simulink subsystem "template_offline_MCP_variant_nlpsol_shared_subsystem"  (R2023b)
settings: Solver=VariableStepAuto  StartTime=0.0  StopTime=10.0  RelTol=1e-3
undefined symbols (not defined in the file): param_MPC1, param_MPC1_traj_data, param_weight_MPC1
settings Model: Creator=emu  LastModifiedBy=emu

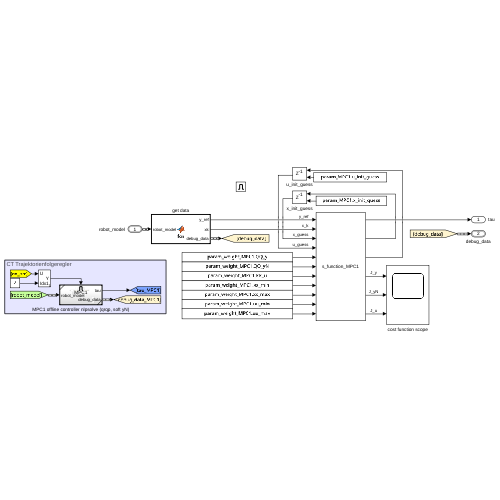
[thumbnail: Simulink's stored preview of the top-level diagram]
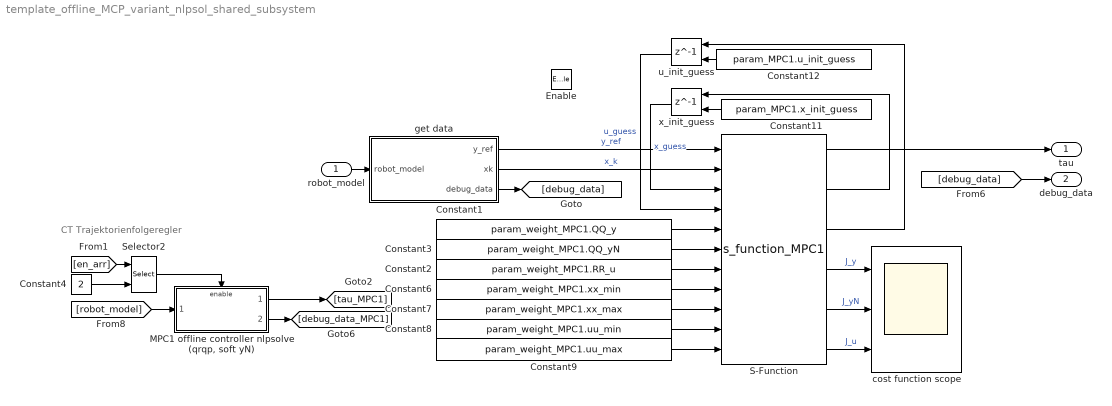
== system template_offline_MCP_variant_nlpsol_shared_subsystem ==
  note: CT Trajektorienfolgeregler
  robot_model : Inport  OutDataTypeStr=Bus: robot_model
  Enable : EnablePort
  Constant1 : Constant  Value=param_weight_MPC1.QQ_y
  Constant11 : Constant  Value=param_MPC1.x_init_guess
  Constant12 : Constant  Value=param_MPC1.u_init_guess
  Constant2 : Constant  Value=param_weight_MPC1.RR_u
  Constant3 : Constant  Value=param_weight_MPC1.QQ_yN
  Constant4 : Constant  Value=2
  Constant6 : Constant  Value=param_weight_MPC1.xx_min
  Constant7 : Constant  Value=param_weight_MPC1.xx_max
  Constant8 : Constant  Value=param_weight_MPC1.uu_min
  Constant9 : Constant  Value=param_weight_MPC1.uu_max
  "MPC1 offline controller nlpsolve (qrqp, soft yN)" : Subsystem  ReferencedSubsystem=MPC1
  S-Function : S-Function  FunctionName=s_function_MPC1  Parameters='s_functions/MPC1.casadi', 'MPC1'  SFunctionDeploymentMode=off  EnableBusSupport=off
  Selector2 : Selector  IndexOptions=Index vector (port)  Indices=[1 3]  OutputSizes=1
  cost function scope : Scope  NumInputPorts=3
  get data : MATLAB Function  TreatAsAtomicUnit=on
  u_init_guess : Delay  DelayLength=1  InitialConditionSource=Input port  InitialCondition=1
      settings: InputPortMap=u0,p4
  x_init_guess : Delay  DelayLength=1  InitialConditionSource=Input port  InitialCondition=1
      settings: InputPortMap=u0,p4
  tau : Outport
  debug_data : Outport  Port=2  OutDataTypeStr=Bus: debug_data_bus
  wires:
  Constant9/1 -> S-Function/11
  get data/1(y_ref) -> S-Function/1  "y_ref"
  S-Function/3 -> u_init_guess/1
  Constant3/1 -> S-Function/6
  Constant6/1 -> S-Function/8
  [debug_data] -> debug_data/1
  u_init_guess/1 -> S-Function/4  "u_guess"
  S-Function/2 -> x_init_guess/1
  Constant11/1 -> x_init_guess/2
  S-Function/4 -> cost function scope/1  "J_y"
  get data/2(xk) -> S-Function/2  "x_k"
  Constant2/1 -> S-Function/7
  Constant12/1 -> u_init_guess/2
  Constant7/1 -> S-Function/9
  Constant8/1 -> S-Function/10
  S-Function/1 -> tau/1
  Constant1/1 -> S-Function/5
  S-Function/6 -> cost function scope/3  "J_u"
  get data/3(debug_data) -> [debug_data]
  S-Function/5 -> cost function scope/2  "J_yN"
  robot_model/1 -> get data/1(robot_model)
  x_init_guess/1 -> S-Function/3  "x_guess"
  "MPC1 offline controller nlpsolve (qrqp, soft yN)"/2 -> [debug_data_MPC1]
  [en_arr] -> Selector2/1
  [robot_model] -> "MPC1 offline controller nlpsolve (qrqp, soft yN)"/1
  Constant4/1 -> Selector2/2
  "MPC1 offline controller nlpsolve (qrqp, soft yN)"/1 -> [tau_MPC1]
  Selector2/1 -> "MPC1 offline controller nlpsolve (qrqp, soft yN)"/Enable

== matlab function template_offline_MCP_variant_nlpsol_shared_subsystem/get data ==
  settings: updateMethod=DISCRETE  sampleTime=param_global.Ta
  data: y_ref output; robot_model input Bus: robot_model; param_MPC1 parameter; xk output; debug_data output Bus: debug_data_bus; param_MPC1_traj_data parameter
function [y_ref, xk, debug_data] = fcn(robot_model, param_MPC1, param_MPC1_traj_data)
persistent cnt;

if(isempty(cnt))
    cnt = 1;
end

param_MPC = param_MPC1;
N = param_MPC.N;
N_step = param_MPC.N_step;
param_trajectory = param_MPC1_traj_data;

% Parameters
q = robot_model.q;      % generalized coordinates
q_p = robot_model.q_p;  % time derivative of generalized coordinates
H = robot_model.H;

% Current Pose of Endeffector
p = H(1:3,4);
R = H(1:3,1:3);

% desired Orientation as Rotationmatrix
q_e = rotation2quaternion(R);

% Error of Position (translation) and first time derivative
q_err = quat_mult(q_e, quat_inv(param_trajectory.q_d(:, cnt)));

xk = [q;q_p];

% Assemble vector of recieved output measurements
p_d_traj = param_trajectory.p_d(1:3, cnt: N_step : cnt + N*N_step);
y_ref = p_d_traj(1:2, 2:N+1);

cnt = cnt+1;

%% DEBUG
debug_data.x = p(1);
debug_data.x_d = p_d_traj(1,1);
debug_data.y =  p(2);
debug_data.y_d = p_d_traj(2,1);
debug_data.z =  p(3);
debug_data.z_d = p_d_traj(3,1);
debug_data.rot_x_err = q_err(2);
debug_data.rot_y_err = q_err(3);
debug_data.rot_z_err = q_err(4);
